simulink model "SMctrl"  (R2018b)
settings: Solver=FixedStepAuto  StartTime=0.0  StopTime=tfin  FixedStep=timeStep  RelTol=1e-3
InitFcn:
  | initSim=true;
  | initSMctrl
StopFcn:
  | initSim=false;
  | initSMctrl
values from neighbouring files (symbols this model uses):
  D = [zeros(6); eye(6)]    [initSMctrl.m]
  KD = diag(kds)    [initSMctrl.m]
  KP = diag(kps)    [initSMctrl.m]
  p = 50    [initSMctrl.m]
  Q = lyap(Htilde',P)    [initSMctrl.m]
libraries: roblocks x4
settings Model: Creator=Brus  LastModifiedBy=Brus

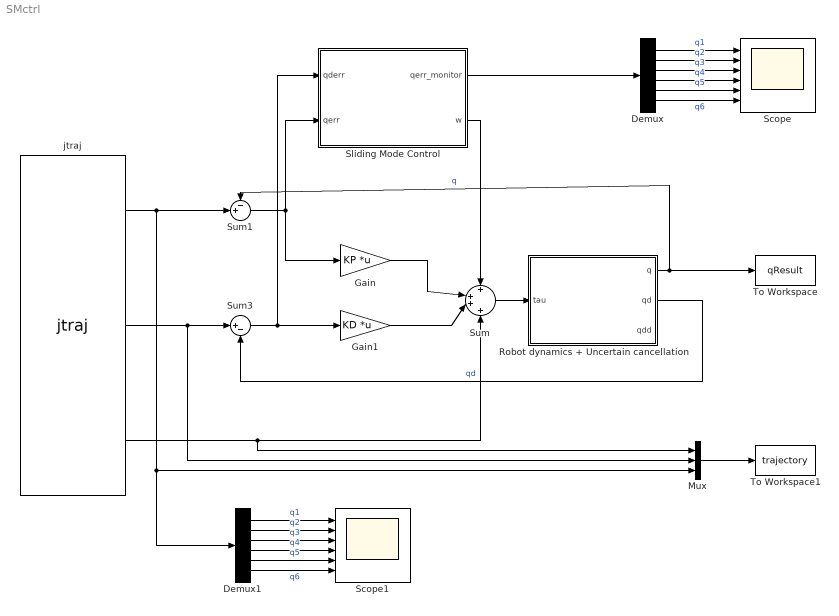
== system SMctrl ==
  Demux : Demux  Outputs=6
  Demux1 : Demux  Outputs=6
  Gain : Gain  Gain=KP  Multiplication=Matrix(K*u)
  Gain1 : Gain  Gain=KD  Multiplication=Matrix(K*u)
  Mux : Mux  Inputs=3
  Robot dynamics + Uncertain cancellation : Subsystem
      mask Display: image('uncArmIcon.png');
  Scope : Scope  NumInputPorts=6
  Scope1 : Scope  NumInputPorts=6
  Sliding Mode Control : Subsystem
      mask Display: image('SMicon.png');
  Sum : Sum  Inputs=+|++|+
  Sum1 : Sum  Inputs=-+|
  Sum3 : Sum  Inputs=|+-
  To Workspace : ToWorkspace  VariableName=qResult  SaveFormat=Timeseries  SampleTime=-1
  To Workspace1 : ToWorkspace  VariableName=trajectory  SaveFormat=Timeseries  SampleTime=-1
  jtraj : roblocks/Toolbox/jtraj  q0=q0  qf=qf  tmax=tfin  ts=timeStep
  wires:
  Sum/1 -> Robot dynamics + Uncertain cancellation/1(tau)
  jtraj/3 -> Mux/1, Sum/4
  Gain/1 -> Sum/2
  Sum3/1 -> Gain1/1, Sliding Mode Control/1(qderr)
  Sum1/1 -> Sliding Mode Control/2(qerr), Gain/1
  jtraj/1 -> Demux1/1, Mux/3, Sum1/2
  Demux/3 -> Scope/3  "q3"
  Demux/6 -> Scope/6  "q6"
  Demux/4 -> Scope/4  "q4"
  Demux/1 -> Scope/1  "q1"
  Demux/2 -> Scope/2  "q2"
  Demux/5 -> Scope/5  "q5"
  Sliding Mode Control/2(w) -> Sum/1
  Robot dynamics + Uncertain cancellation/1(q) -> To Workspace/1, Sum1/1  "q"
  Robot dynamics + Uncertain cancellation/2(qd) -> Sum3/2  "qd"
  Gain1/1 -> Sum/3
  jtraj/2 -> Mux/2, Sum3/1
  Mux/1 -> To Workspace1/1
  Demux1/6 -> Scope1/6  "q6"
  Demux1/2 -> Scope1/2  "q2"
  Demux1/4 -> Scope1/4  "q4"
  Demux1/1 -> Scope1/1  "q1"
  Demux1/5 -> Scope1/5  "q5"
  Demux1/3 -> Scope1/3  "q3"
  Sliding Mode Control/1(qerr_monitor) -> Demux/1

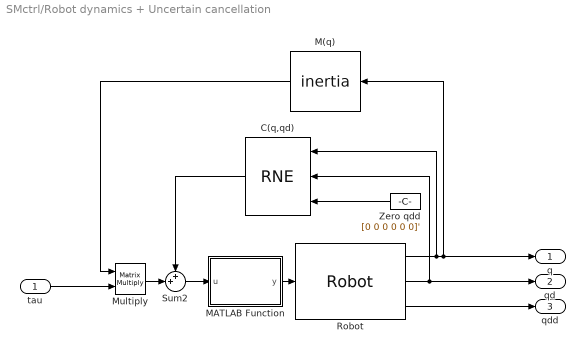
== system SMctrl/Robot dynamics + Uncertain cancellation ==
  tau : Inport
  C(q,qd) : roblocks/Arm/RNE  robot=p560Unc  grav=[0 0 9.81]
  M(q) : roblocks/Arm/inertia  robot=p560Unc
  MATLAB Function : MATLAB Function  TreatAsAtomicUnit=on
  Multiply : Product  Multiplication=Matrix(*)
  Robot : roblocks/Arm/Robot  robot=p560  q0=q0
  Sum2 : Sum  Inputs=++|
  Zero qdd : Constant  Value=[0 0 0 0 0 0]'
  q : Outport
  qd : Outport  Port=2
  qdd : Outport  Port=3
  wires:
  Multiply/1 -> Sum2/2
  Robot/3 -> qdd/1
  Zero qdd/1 -> C(q,qd)/3
  M(q)/1 -> Multiply/1
  Sum2/1 -> MATLAB Function/1(u)
  MATLAB Function/1(y) -> Robot/1
  C(q,qd)/1 -> Sum2/1
  Robot/2 -> C(q,qd)/2, qd/1
  Robot/1 -> M(q)/1, q/1, C(q,qd)/1
  tau/1 -> Multiply/2

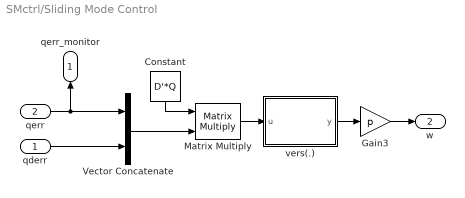
== system SMctrl/Sliding Mode Control ==
  qderr : Inport
  qerr : Inport  Port=2
  Constant : Constant  Value=D'*Q
  Gain3 : Gain  Gain=p
  Matrix Multiply : Product  Multiplication=Matrix(*)
  Vector Concatenate : Concatenate  Mode=Multidimensional array
  vers(.) : MATLAB Function  TreatAsAtomicUnit=on
  qerr_monitor : Outport
  w : Outport  Port=2
  wires:
  Constant/1 -> Matrix Multiply/1
  Vector Concatenate/1 -> Matrix Multiply/2
  qerr/1 -> qerr_monitor/1, Vector Concatenate/1
  qderr/1 -> Vector Concatenate/2
  Matrix Multiply/1 -> vers(.)/1(u)
  vers(.)/1(y) -> Gain3/1
  Gain3/1 -> w/1

== matlab function SMctrl/Robot dynamics + Uncertain cancellation/MATLAB Function ==
  data: u input; y output
function y = checkNaN(u)
if(isnan(u))
    y=zeros(size(u));
else
    y=u;
end

== matlab function SMctrl/Sliding Mode Control/vers(.) ==
  data: u input; y output
function y = vers(u)

y = vers(u);
